simulink model "longSim"  (R2023a)
settings: Solver=VariableStepAuto  StartTime=0.0  StopTime=1000  RelTol=1e-3
settings Model: Creator=User  LastModifiedBy=User

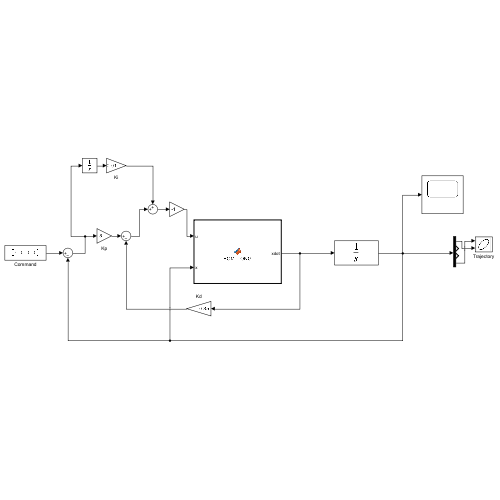
[thumbnail: Simulink's stored preview of the top-level diagram]
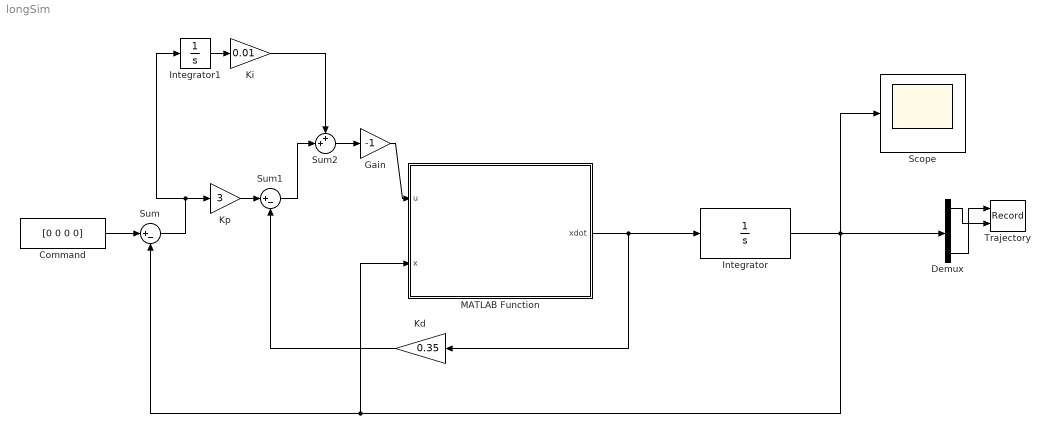
== system longSim ==
  Command : Constant  Value=[0 0 0 0]
  Demux : Demux
  Gain : Gain  Gain=-1
  Integrator : Integrator  InitialCondition=[0; 0; 1*(pi/180); 1*(pi/180)]
  Integrator1 : Integrator
  Kd : Gain  Gain=0.35
  Ki : Gain  Gain=0.01
  Kp : Gain  Gain=3
  MATLAB Function : MATLAB Function  TreatAsAtomicUnit=on
  Scope : Scope
  Sum : Sum  Inputs=|+-
  Sum1 : Sum  Inputs=|+-
  Sum2 : Sum  Inputs=++|
  Trajectory : Record  FileSettingsInternal="{\"entries\":[{\"content\":{\"excelSettings\":{\"content\":{},\"type\":\"Streamout.ExcelSettings\"}},\"type\":\"Streamout.FileSettingStorage\",\"uuid\":\"7b14ae47-46ac-4e09-858c-777531cd8c47\"}],\"packageUris\":[\"http://schema.mathworks.com/mf0/streamout_blocks/R2020a\"],\"version\":\"1.0\"}"  Layout=[1 2]  SignalsInternal="{\"entries\":[{\"content\":{\"signals\":[{\"content\":{\"blockPath\":[\"untitled1/Trajectory\"],\"dimensions\":[1,1],\"domain\":\"untitled1/Trajectory\",\"lineColor\":\"#a2142f\",\"plots\":[1],\"port\":1,\"sid\":[\"\"],\"signalID\":647,\"signalName\":\"Demux:4\"},\"type\":\"RecordBlkView.Signal\",\"uuid\":\"7885491d-e779-441b-b65c-d3df47f2229a\"},{\"content\":{\"blockPath\":[\"untitled1/Trajectory\"],\"dimensions\":[1,1],\"domain\":\"untitled1/Trajectory\",\"lineColor\":\"#139fff\",\"plots\":[1],\"port\":2,\"sid\":[\"\"],\"signalID\":651,\"signalName\":\"Demux:1\"},\"type\":\"RecordBlkView.Signal\",\"uuid\":\"186fea7e-6d7f-480f-88db-2cd894a9a0bb\"}]},\"type\":\"RecordBlkView.InputSignals\",\"uuid\":\"cc9dff25-82d2-4ddb-b54f-be46748c88a2\"}],\"packageUris\":[\"http://schema.mathworks.com/mf0/streamout_blocks/R2020a\"],\"version\":\"1.0\"}"  VisualizationBindings="{\"xyplotplugin\":{\"info\":[{\"series\":[],\"subplotID\":1}]}}"  CompatibilityTag=XY
  wires:
  Integrator/1 -> MATLAB Function/2(x), Sum/2, Demux/1, Scope/1
  MATLAB Function/1(xdot) -> Kd/1, Integrator/1
  Sum/1 -> Kp/1, Integrator1/1
  Command/1 -> Sum/1
  Kp/1 -> Sum1/1
  Kd/1 -> Sum1/2
  Sum1/1 -> Sum2/2
  Gain/1 -> MATLAB Function/1(u)
  Demux/4 -> Trajectory/1
  Demux/1 -> Trajectory/2
  Integrator1/1 -> Ki/1
  Ki/1 -> Sum2/1
  Sum2/1 -> Gain/1

== matlab function longSim/MATLAB Function ==
  data: u input; x input; xdot output
function xdot = EOM_LONG(u, x)

%% Initial Mass & Geometry Properties
%Givens
W = 6360; %lb
g = 32.2; %ft/s2
Ixx = 7.99e3; %slug ft2
Iyy = 3.33e3; %slug ft2
Izz = 1.12e4; %slug ft2
Ixz = -3.91e1; %slug ft2

m = W/32.2; %lb

%Inertial Matrix
I = [Ixx, 0,-Ixz;
      0, Iyy, 0;
    -Ixz, 0, Izz]; 

S = 182; %ft2
b = 33.8; %ft
c_hat = 5.47; %ft
x_cg = 27; 
trim_aoa = 0; %deg

%% Longitudinal Derivatives
Xu = -0.0168;
Xa = 14.8205;
Zu = -0.1844;
Za = -645.1571;
Mu = 0;
Ma = -28.9722;
Madot = -2.2569;
Mq = -4.8604;
Xde = 0;
Zde = -53.4070;
Mde = -46.4075;
theta = trim_aoa*(pi/180);
U1 = 349;

%% Mapping Out Longitudinal Motion
%unpack state from the q state column vector
x = x(1:4);

%******** Motion *************
A1 = [        Xu                 Xa                   0         -g*cos(theta);
            Zu/U1               Za/U1                1        (-g*sin(theta)/U1);
      Mu + (Madot/U1)*Zu  Ma + Madot*(Za/U1)     Mq + Madot         0;
             0                  0                    1              0];


%******** Control *************
B1 = [    Xde;
         Zde/U1;
      Mde + (Madot/U1)*Zde;
           0];
u = u(4);

xdot = A1*x + B1*u;
end
